simulink model "reference"  (R2017b)
settings: Solver=ode4  StartTime=0.0  StopTime=1.2  FixedStep=1e-6  RelTol=1e-3
values from neighbouring files (symbols this model uses):
  Vdc = 36    [ParameterInit.m]    (also in parameter_init.m)
undefined symbols (not defined in the file or in its folder): sigbuilder_block
libraries: powerlib x9, peTransforms x2, powerlib_meascontrol x1
settings Model: Creator=Admin  LastModifiedBy=Admin
settings DataIOCC: ReturnWorkspaceOutputs=on
settings OptimizationCC: LifeSpan=inf
settings DebuggingCC: SFExecutionAtInitializationDiag=none
settings SFSimCC: SimUseLocalCustomCode=on
settings RTWCC: RTWUseLocalCustomCode=on
settings CodeAppCC: StateflowObjectComments=on

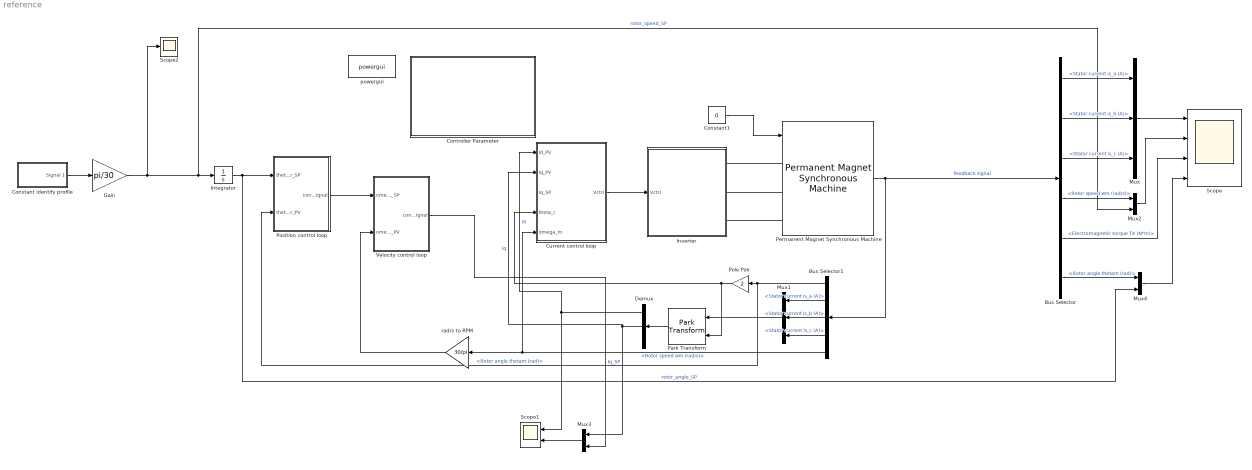
== system reference ==
  Bus Selector : BusSelector  OutputSignals=Stator current is_a (A),Stator current is_b (A),Stator current is_c (A),Rotor speed wm (rad/s),Electromagnetic torque Te (N*m),Rotor angle thetam (rad)
  Bus Selector1 : BusSelector  OutputSignals=Rotor angle thetam (rad),Stator current is_a (A),Stator current is_b (A),Stator current is_c (A),Rotor speed wm (rad/s)
  Constant identify profile : Subsystem  Tag=STV Subsys  LoadFcn=sigbuilder_block('load');  StartFcn=sigbuilder_block('start');  StopFcn=sigbuilder_block('stop');  ClipboardFcn=sigbuilder_block('clipboard');  mask(Sigbuilder block){tuvar=[0:10]}
      mask help: Simulink:masks:SigbuilderBlock_MD
      mask init:
      | if ~strcmp(get_param(bdroot(gcbh),'SimulationStatus'),'stopped') tuvar = sigbuilder_block('maskInit'); end
      settings: CopyFcn=sigbuilder_block('copy');  DeleteFcn=sigbuilder_block('delete');  ModelCloseFcn=sigbuilder_block('modelClose');  PreSaveFcn=sigbuilder_block('preSave');  PauseFcn=sigbuilder_block('pause');  ContinueFcn=sigbuilder_block('continue');  NameChangeFcn=sigbuilder_block('namechange');  OpenFcn=sigbuilder_block('open',[356.4 94.8 550.8 400.2 ]);  CloseFcn=sigbuilder_block('close');
      mask Display: plot(0, 0, 100, 100,[2, 2, 32, 32, 2], [68, 8, 8, 68, 68],[32, 2], [38, 38], [32, 19, 2],[53, 60, 44], [32, 17, 17, 2],[16, 16, 31, 31]);txt = getActiveGroup(gcbh);text(2, 100, txt,'verticalAlignment', 'top');
  Constant1 : Constant  Value=0
  Controller Parameter : Subsystem  mask{PID_Id=[1200 800 0], PID_Iq=[1200 800 0], PID_velocity=[0.015 0.04 0], PID_position=[100 0 0]}
      mask prompts: PID_Id "PID param Id"; PID_Iq "PID param Iq"; PID_velocity "PID param velocity"; PID_position "PID param position"
  Current control loop : Subsystem  mask{Ld=0.02682, Lq=0.02682, psi_m=0.1716}
      mask prompts: Ld "Độ tự cảm trục d"; Lq "Độ tự cảm trục q"; psi_m "Liên kết từ thông NCVC"
  Demux : Demux  Outputs=3
  Gain : Gain  Gain=pi/30
  Integrator : Integrator
  "Inverter " : Subsystem
  Mux : Mux  Inputs=3
  Mux1 : Mux  Inputs=3
  Mux2 : Mux  Inputs=2
  Mux3 : Mux  Inputs=2
  Mux4 : Mux  Inputs=2
  Park Transform : peTransforms/Park Transform  AxisAlignment=Q-axis  PowerInvariant=off
  Permanent Magnet Synchronous Machine : powerlib/Machines/Permanent Magnet Synchronous Machine  NbPhases=3  FluxDistribution=Sinusoidal  RotorType=Round  MechanicalLoad=Torque Tm  PresetModel="01:  0.8 Nm 300 Vdc 3000 RPM - 0.8 Nm"  ShowDetailedParameters=on  MeasurementBus=off  Resistance=18.7  Inductance=8.5e-3  dqInductances=[8.5e-3,8.5e-3]  La=0.02682  MachineConstant=Flux linkage established by magnets (V.s)  Flux=0.1716  VoltageCst=62.2496  TorqueCst=0.5148  Flat=120  Mechanical=[2.26e-05 1.349e-05 2 0]  PolePairs=2  InitialConditions=[0,0, 0,0]  InitialConditions5ph=[0 0 0 0 0 0]  TsPowergui=0  TsBlock=-1  RefAngle=90 degrees behind phase A axis (modified Park)
      settings: SourceProductName=Simscape Power Systems
  Pole Pair : Gain  Gain=2
  Position control loop : Subsystem
  Scope : Scope  NumInputPorts=4
  Scope1 : Scope  NumInputPorts=2
  Scope2 : Scope
  Velocity control loop : Subsystem
  powergui : powerlib/powergui  Priority=1  SimulationMode=Discrete  SampleTime=1e-6  frequency=60  Iterations=50  frequencyindice=0  Pbase=100e6  ErrMax=1e-4  UnitsV=kV  UnitsW=MW  buscounter=0  FunctionMessages=off  echomessages=off  EnableUseOfTLC=off  CurrentSourceSwitches=off  DisableSnubberDevices=off  DisableRonSwitches=off  DisableVfSwitches=off  DisplayEquations=off  SolverType=Tustin/Backward Euler (TBE)  Interpol=off  ExternalGateDelay=off  methode=off  Ts=100  x0status=blocks  SPID=on  SwTol=0  HookPort=off  RestoreLinks=warning  ResistiveCurrentMeasurement=off  Frange=[0:2:500]  Ylog=off  Xlog=on  ShowGrid=off  save=off  variable=ZData  structure=0  ZoomFFT=off  StartTime=0.0  cycles=1  DisplayStyle=1  fundamental=60  FreqAxis=off  MaxFrequency=1000  frequencyindicesteady=1  RmsSteady=1  display=off
  rad/s to RPM : Gain  Gain=30/pi
  wires:
  Bus Selector/1 -> Mux/1  "<Stator current is_a (A)>"
  Mux/1 -> Scope/1
  Permanent Magnet Synchronous Machine/1 -> Bus Selector1/1, Bus Selector/1  "feedback signal"
  Bus Selector/2 -> Mux/2  "<Stator current is_b (A)>"
  Bus Selector/3 -> Mux/3  "<Stator current is_c (A)>"
  Current control loop/1(Vctrl) -> "Inverter "/1(Vctrl)
  Bus Selector/5 -> Scope/3  "<Electromagnetic torque Te (N*m)>"
  Mux1/1 -> Park Transform/1
  Park Transform/1 -> Demux/1
  Bus Selector1/2 -> Mux1/1  "<Stator current is_a (A)>"
  Bus Selector1/3 -> Mux1/2  "<Stator current is_b (A)>"
  Bus Selector1/4 -> Mux1/3  "<Stator current is_c (A)>"
  Pole Pair/1 -> Park Transform/2, Current control loop/4(theta_r)
  Demux/1 -> Scope1/1, Current control loop/1(Id_PV)  "Id"
  Demux/2 -> Mux3/1, Current control loop/2(Iq_PV)  "Iq"
  Bus Selector1/5 -> Current control loop/5("omega_m "), rad/s to RPM/1  "<Rotor speed wm (rad/s)>"
  rad/s to RPM/1 -> Velocity control loop/2(omega_PV)
  Integrator/1 -> Mux4/2, Position control loop/1("theta_rotor_SP ")  "rotor_angle_SP"
  Bus Selector/4 -> Mux2/1  "<Rotor speed wm (rad/s)>"
  Mux2/1 -> Scope/2
  Mux3/1 -> Scope1/2
  Gain/1 -> Scope2/1, Mux2/2, Integrator/1  "rotor_speed_SP"
  Position control loop/1(control signal) -> Velocity control loop/1("omega_SP ")
  Velocity control loop/1(control signal) -> Mux3/2  "Iq_SP"
  Bus Selector/6 -> Mux4/1  "<Rotor angle thetam (rad)>"
  Mux4/1 -> Scope/4
  Constant1/1 -> Permanent Magnet Synchronous Machine/1
  Bus Selector1/1 -> Position control loop/2(theta_rotor_PV), Pole Pair/1  "<Rotor angle thetam (rad)>"
  Constant identify profile/1(Signal 1) -> Gain/1
  connections:
  Permanent Magnet Synchronous Machine/LConn1 -- "Inverter "/RConn1
  Permanent Magnet Synchronous Machine/LConn2 -- "Inverter "/RConn2
  Permanent Magnet Synchronous Machine/LConn3 -- "Inverter "/RConn3

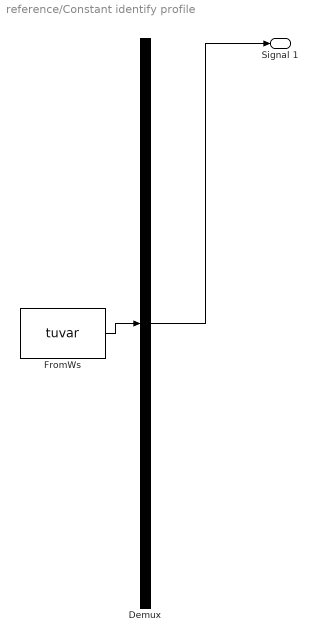
== system reference/Constant identify profile ==
  Demux : Demux  Tag=STV Demux  Outputs=1
  FromWs : FromWorkspace  Tag=STV FromWs  VariableName=tuvar  SampleTime=0
      SigBuilderData=|
      | common.afterFinalStr = 'Extrapolate'
      | common.sampleTime = 0
      | dataSet.timeRange = [0 1.2]
      | dataSet.name = 'Group 1'
      | sbobj.Groups.Name = 'Group 1'
      | sbobj.Groups.Signals.Name = 'Signal 1'
      | sbobj.Groups.Signals.XData = [0 0.2 0.6 0.8 1.2]
      | sbobj.Groups.Signals.YData = [0.005 100 100 0 0.005]
      | sbobj.Groups.TimeRange = [0 1.2]
  Signal 1 : Outport  Tag=STV Outport
  wires:
  Demux/1 -> Signal 1/1
  FromWs/1 -> Demux/1

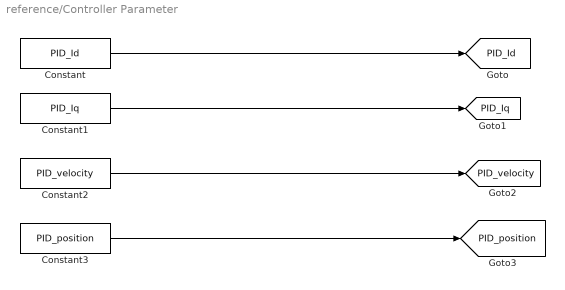
== system reference/Controller Parameter ==
  Constant : Constant  Value=PID_Id
  Constant1 : Constant  Value=PID_Iq
  Constant2 : Constant  Value=PID_velocity
  Constant3 : Constant  Value=PID_position
  tag scope: PID_Id=global, PID_Iq=global, PID_position=global, PID_velocity=global
  wires:
  Constant/1 -> [PID_Id]
  Constant1/1 -> [PID_Iq]
  Constant2/1 -> [PID_velocity]
  Constant3/1 -> [PID_position]

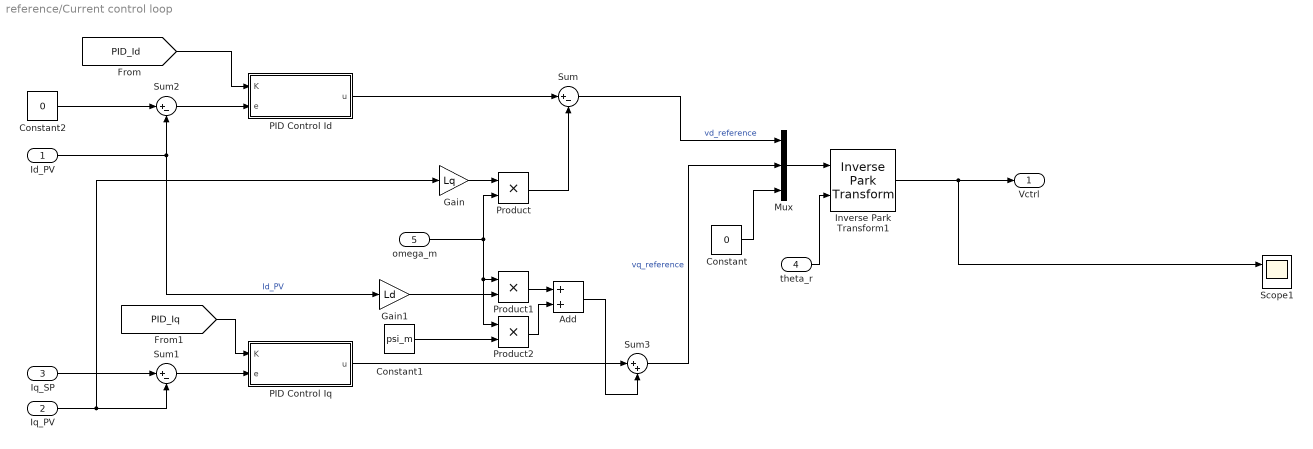
== system reference/Current control loop ==
  Id_PV : Inport
  Iq_PV : Inport  Port=2
  Iq_SP : Inport  Port=3
  theta_r : Inport  Port=4
  "omega_m " : Inport  Port=5
  Add : Sum
  Constant : Constant  Value=0
  Constant1 : Constant  Value=psi_m
  Constant2 : Constant  Value=0
  Gain : Gain  Gain=Lq
  Gain1 : Gain  Gain=Ld
  Inverse Park Transform1 : peTransforms/Inverse Park Transform  AxisAlignment=Q-axis  PowerInvariant=off
  Mux : Mux  Inputs=3
  PID Control Id : Subsystem
  PID Control Iq : Subsystem
  Product : Product
  Product1 : Product
  Product2 : Product
  Scope1 : Scope  NumInputPorts=2
  Sum : Sum  Inputs=|+-
  Sum1 : Sum  Inputs=|+-
  Sum2 : Sum  Inputs=|+-
  Sum3 : Sum  Inputs=|++
  Vctrl : Outport
  wires:
  Id_PV/1 -> Gain1/1, Sum2/2  "Id_PV"
  Iq_PV/1 -> Sum1/2, Gain/1
  Iq_SP/1 -> Sum1/1
  Sum2/1 -> PID Control Id/2(e)
  Sum1/1 -> PID Control Iq/2(e)
  Mux/1 -> Inverse Park Transform1/1
  theta_r/1 -> Inverse Park Transform1/2
  [PID_Iq] -> PID Control Iq/1(K)
  Constant/1 -> Mux/3
  [PID_Id] -> PID Control Id/1(K)
  PID Control Id/1(u) -> Sum/1
  Gain/1 -> Product/1
  "omega_m "/1 -> Product2/1, Product1/1, Product/2
  Product/1 -> Sum/2
  Sum/1 -> Mux/1  "vd_reference"
  PID Control Iq/1(u) -> Sum3/1
  Sum3/1 -> Mux/2  "vq_reference"
  Gain1/1 -> Product1/2
  Product1/1 -> Add/1
  Product2/1 -> Add/2
  Constant1/1 -> Product2/2
  Add/1 -> Sum3/2
  Constant2/1 -> Sum2/1
  Inverse Park Transform1/1 -> Scope1/1, Vctrl/1

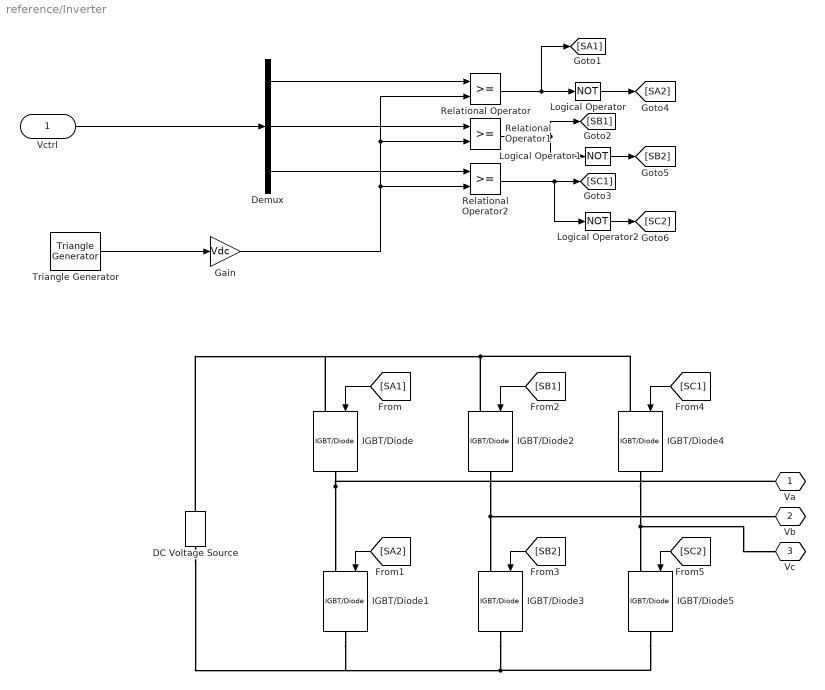
== system reference/Inverter  ==
  Vctrl : Inport
  DC Voltage Source : powerlib/Electrical Sources/DC Voltage Source  Amplitude=Vdc  Measurements=None
  Demux : Demux  Outputs=3
  Gain : Gain  Gain=Vdc
  IGBT/Diode{,1..5} (6 alike) : powerlib/Power Electronics/IGBT//Diode  Ron=1e-3  Rs=1e5  Cs=inf  Measurements=off
  Logical Operator : Logic  Operator=NOT  AllPortsSameDT=off  OutDataTypeStr=boolean
  Logical Operator1 : Logic  Operator=NOT  AllPortsSameDT=off  OutDataTypeStr=boolean
  Logical Operator2 : Logic  Operator=NOT  AllPortsSameDT=off  OutDataTypeStr=boolean
  Relational Operator : RelationalOperator  OutDataTypeStr=boolean  RndMeth=Nearest
  Relational Operator1 : RelationalOperator  OutDataTypeStr=boolean  RndMeth=Nearest
  Relational Operator2 : RelationalOperator  OutDataTypeStr=boolean  RndMeth=Nearest
  Triangle Generator : powerlib_meascontrol/Pulse & Signal Generators/Triangle Generator  Freq=20000  Phase=90  Ts=1e-6
  Va : PMIOPort  Tag=PMCPort  Port=1  Side=Right
  Vb : PMIOPort  Tag=PMCPort  Port=2  Side=Right
  Vc : PMIOPort  Tag=PMCPort  Port=3  Side=Right
  wires:
  [SB2] -> IGBT/Diode3/1
  [SA1] -> IGBT/Diode/1
  [SB1] -> IGBT/Diode2/1
  [SC2] -> IGBT/Diode5/1
  [SC1] -> IGBT/Diode4/1
  [SA2] -> IGBT/Diode1/1
  Logical Operator2/1 -> [SC2]
  Logical Operator1/1 -> [SB2]
  Logical Operator/1 -> [SA2]
  Relational Operator2/1 -> Logical Operator2/1, [SC1]
  Demux/1 -> Relational Operator/1
  Demux/3 -> Relational Operator2/1
  Demux/2 -> Relational Operator1/1
  Relational Operator/1 -> [SA1], Logical Operator/1
  Relational Operator1/1 -> Logical Operator1/1, [SB1]
  Triangle Generator/1 -> Gain/1
  Vctrl/1 -> Demux/1
  Gain/1 -> Relational Operator2/2, Relational Operator1/2, Relational Operator/2
  connections:
  IGBT/Diode2/LConn1 -- IGBT/Diode4/LConn1 -- DC Voltage Source/RConn1 -- IGBT/Diode/LConn1
  IGBT/Diode4/RConn1 -- IGBT/Diode5/LConn1 -- Vc/RConn1
  IGBT/Diode/RConn1 -- IGBT/Diode1/LConn1 -- Va/RConn1
  IGBT/Diode3/RConn1 -- DC Voltage Source/LConn1 -- IGBT/Diode1/RConn1 -- IGBT/Diode5/RConn1
  IGBT/Diode2/RConn1 -- Vb/RConn1 -- IGBT/Diode3/LConn1

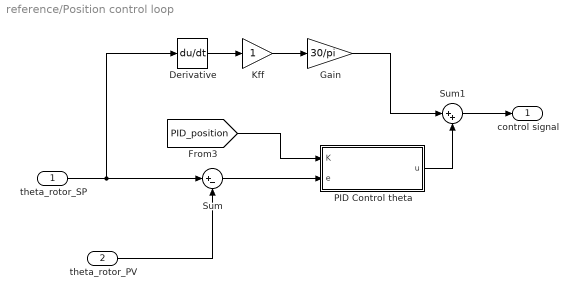
== system reference/Position control loop ==
  "theta_rotor_SP " : Inport
  theta_rotor_PV : Inport  Port=2
  Derivative : Derivative
  Gain : Gain  Gain=30/pi
  Kff : Gain
  PID Control theta : Subsystem
  Sum : Sum  Inputs=|+-
  Sum1 : Sum  Inputs=|++
  control signal : Outport
  wires:
  "theta_rotor_SP "/1 -> Derivative/1, Sum/1
  theta_rotor_PV/1 -> Sum/2
  Sum/1 -> PID Control theta/2(e)
  [PID_position] -> PID Control theta/1(K)
  Derivative/1 -> Kff/1
  PID Control theta/1(u) -> Sum1/2
  Sum1/1 -> control signal/1
  Kff/1 -> Gain/1
  Gain/1 -> Sum1/1

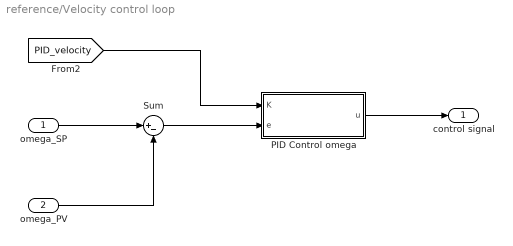
== system reference/Velocity control loop ==
  "omega_SP " : Inport
  omega_PV : Inport  Port=2
  PID Control omega : Subsystem
  Sum : Sum  Inputs=|+-
  control signal : Outport
  wires:
  "omega_SP "/1 -> Sum/1
  omega_PV/1 -> Sum/2
  Sum/1 -> PID Control omega/2(e)
  PID Control omega/1(u) -> control signal/1
  [PID_velocity] -> PID Control omega/1(K)

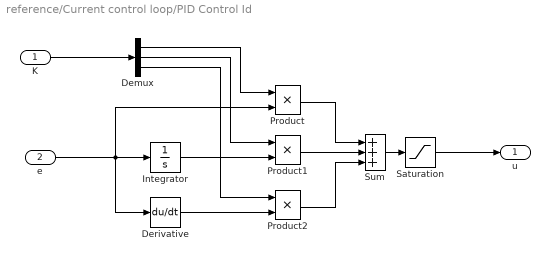
== system reference/Current control loop/PID Control Id ==
  K : Inport
  e : Inport  Port=2
  Demux : Demux  Outputs=3
  Derivative : Derivative
  Integrator : Integrator
  Product : Product  SaturateOnIntegerOverflow=on  OutDataTypeStr=Inherit: Same as first input
  Product1 : Product  SaturateOnIntegerOverflow=on  OutDataTypeStr=Inherit: Same as first input
  Product2 : Product  SaturateOnIntegerOverflow=on  OutDataTypeStr=Inherit: Same as first input
  Saturation : Saturate  UpperLimit=200  LowerLimit=-200
  Sum : Sum  Inputs=+++  SaturateOnIntegerOverflow=on  InputSameDT=on  OutDataTypeStr=Inherit: Same as first input
  u : Outport
  wires:
  Demux/2 -> Product1/1
  Demux/1 -> Product/1
  Demux/3 -> Product2/1
  e/1 -> Product/2, Integrator/1, Derivative/1
  Product2/1 -> Sum/3
  Integrator/1 -> Product1/2
  Derivative/1 -> Product2/2
  Product/1 -> Sum/1
  K/1 -> Demux/1
  Product1/1 -> Sum/2
  Sum/1 -> Saturation/1
  Saturation/1 -> u/1

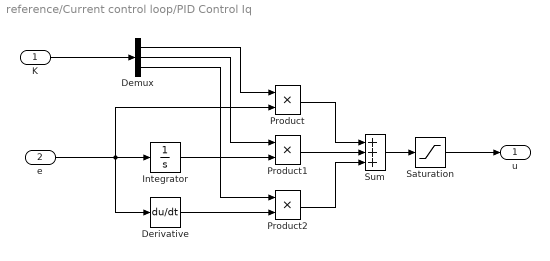
== system reference/Current control loop/PID Control Iq ==
  K : Inport
  e : Inport  Port=2
  Demux : Demux  Outputs=3
  Derivative : Derivative
  Integrator : Integrator
  Product : Product  SaturateOnIntegerOverflow=on  OutDataTypeStr=Inherit: Same as first input
  Product1 : Product  SaturateOnIntegerOverflow=on  OutDataTypeStr=Inherit: Same as first input
  Product2 : Product  SaturateOnIntegerOverflow=on  OutDataTypeStr=Inherit: Same as first input
  Saturation : Saturate  UpperLimit=200  LowerLimit=-200
  Sum : Sum  Inputs=+++  SaturateOnIntegerOverflow=on  InputSameDT=on  OutDataTypeStr=Inherit: Same as first input
  u : Outport
  wires:
  Demux/2 -> Product1/1
  Demux/1 -> Product/1
  Demux/3 -> Product2/1
  e/1 -> Product/2, Integrator/1, Derivative/1
  Product2/1 -> Sum/3
  Integrator/1 -> Product1/2
  Derivative/1 -> Product2/2
  Product/1 -> Sum/1
  K/1 -> Demux/1
  Product1/1 -> Sum/2
  Sum/1 -> Saturation/1
  Saturation/1 -> u/1

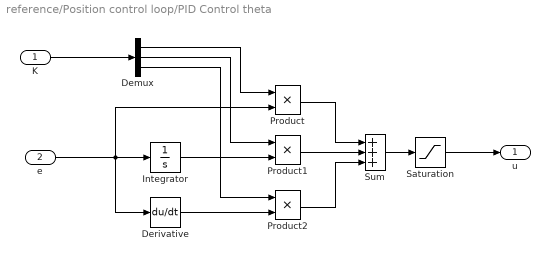
== system reference/Position control loop/PID Control theta ==
  K : Inport
  e : Inport  Port=2
  Demux : Demux  Outputs=3
  Derivative : Derivative
  Integrator : Integrator
  Product : Product  SaturateOnIntegerOverflow=on  OutDataTypeStr=Inherit: Same as first input
  Product1 : Product  SaturateOnIntegerOverflow=on  OutDataTypeStr=Inherit: Same as first input
  Product2 : Product  SaturateOnIntegerOverflow=on  OutDataTypeStr=Inherit: Same as first input
  Saturation : Saturate  UpperLimit=12  LowerLimit=-12
  Sum : Sum  Inputs=+++  SaturateOnIntegerOverflow=on  InputSameDT=on  OutDataTypeStr=Inherit: Same as first input
  u : Outport
  wires:
  Demux/2 -> Product1/1
  Demux/1 -> Product/1
  Demux/3 -> Product2/1
  e/1 -> Product/2, Integrator/1, Derivative/1
  Product2/1 -> Sum/3
  Integrator/1 -> Product1/2
  Derivative/1 -> Product2/2
  Product/1 -> Sum/1
  Sum/1 -> Saturation/1
  K/1 -> Demux/1
  Product1/1 -> Sum/2
  Saturation/1 -> u/1

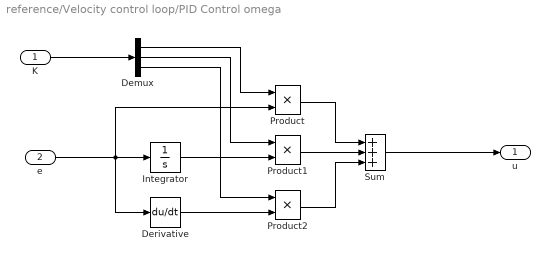
== system reference/Velocity control loop/PID Control omega ==
  K : Inport
  e : Inport  Port=2
  Demux : Demux  Outputs=3
  Derivative : Derivative
  Integrator : Integrator
  Product : Product  SaturateOnIntegerOverflow=on  OutDataTypeStr=Inherit: Same as first input
  Product1 : Product  SaturateOnIntegerOverflow=on  OutDataTypeStr=Inherit: Same as first input
  Product2 : Product  SaturateOnIntegerOverflow=on  OutDataTypeStr=Inherit: Same as first input
  Sum : Sum  Inputs=+++  SaturateOnIntegerOverflow=on  InputSameDT=on  OutDataTypeStr=Inherit: Same as first input
  u : Outport
  wires:
  Demux/2 -> Product1/1
  Demux/1 -> Product/1
  Demux/3 -> Product2/1
  e/1 -> Product/2, Integrator/1, Derivative/1
  Product2/1 -> Sum/3
  Integrator/1 -> Product1/2
  Derivative/1 -> Product2/2
  Product/1 -> Sum/1
  K/1 -> Demux/1
  Product1/1 -> Sum/2
  Sum/1 -> u/1
